simulink model "simu_lqr2"  (R2018b)
settings: Solver=VariableStepAuto  StartTime=0.0  StopTime=7  RelTol=1e-3
values from neighbouring files (symbols this model uses):
  A = [                        0, 1, 0,                0 ... (first row only)    [sistema.m]
  B = [0; (-L*m*p1)/(M+m); 0; p2]    [sistema.m]
  C = eye(4)    [sistema.m]
  D = zeros(4,1)    [sistema.m]
  x0 = [0.2; 0; 0; 0]    [sistema.m]
undefined symbols (not defined in the file or in its folder): K
settings Model: Creator=vuvux  LastModifiedBy=vuvux

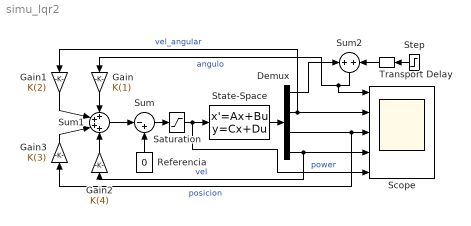
== system simu_lqr2 ==
  Demux : Demux
  Gain : Gain  Gain=K(1)
      settings: AttributesFormatString=%<Gain>
  Gain1 : Gain  Gain=K(2)
      settings: AttributesFormatString=%<Gain>
  Gain2 : Gain  Gain=K(4)
      settings: AttributesFormatString=%<Gain>
  Gain3 : Gain  Gain=K(3)
      settings: AttributesFormatString=%<Gain>
  Referencia : Constant  Value=0
  Saturation : Saturate  UpperLimit=5  LowerLimit=-5
  Scope : Scope  NumInputPorts=5
  State-Space : StateSpace  A=A  B=B  C=C  D=D  InitialCondition=x0
  Step : Step  Before=0.1  After=0  SampleTime=0
  Sum : Sum  Inputs=|-+
  Sum1 : Sum  Inputs=++++
  Sum2 : Sum
  Transport Delay : TransportDelay  DelayTime=4
  wires:
  State-Space/1 -> Demux/1
  Demux/4 -> Scope/4, Gain2/1  "vel"
  Demux/1 -> Sum2/1
  Demux/2 -> Scope/2, Gain1/1  "vel_angular"
  Demux/3 -> Gain3/1, Scope/3  "posicion"
  Sum/1 -> Saturation/1
  Sum1/1 -> Sum/1
  Referencia/1 -> Sum/2
  Gain/1 -> Sum1/1
  Gain1/1 -> Sum1/2
  Gain2/1 -> Sum1/4
  Gain3/1 -> Sum1/3
  Saturation/1 -> Scope/5, State-Space/1  "power"
  Transport Delay/1 -> Sum2/2
  Step/1 -> Transport Delay/1
  Sum2/1 -> Gain/1, Scope/1  "angulo"
